simulink model "semaphore_0"  (R2024b)
settings: Solver=FixedStepDiscrete  StartTime=0.0  StopTime=inf  FixedStep=0.1  RelTol=1e-3
settings Model: PacingRate=0.040000  Creator=Gennaro  LastModifiedBy=miche
settings OptimizationCC: DefaultParameterBehavior=Inlined  UseDivisionForNetSlopeComputation=on  GainParamInheritBuiltInType=on  UseFloatMulNetSlope=on  InlineInvariantSignals=on  PassReuseOutputArgsAs=Individual arguments  ZeroExternalMemoryAtStartup=off  ZeroInternalMemoryAtStartup=off  NoFixptDivByZeroProtection=on  EfficientFloat2IntCast=on  LifeSpan=1  OptimizeBlockOrder=speed  DifferentSizesBufferReuse=on  EfficientTunableParamExpr=on
settings DebuggingCC: ParameterTunabilityLossMsg=error
settings HardwareCC: ProdBitPerPointer=32  ProdBitPerSizeT=32  ProdBitPerPtrDiffT=32  ProdLargestAtomicInteger=Long  ProdLargestAtomicFloat=Double  ProdWordSize=32  ProdLongLongMode=on  ProdHWDeviceType=ARM Compatible->ARM Cortex-M
settings SFSimCC: MATLABDynamicMemAlloc=off
settings RTWCC: Description=Embedded Coder  SystemTargetFile=ert.tlc  TemplateMakefile=ert_default_tmf
settings CodeAppCC: ForceParamTrailComments=on  IgnoreCustomStorageClasses=off  OperatorAnnotations=on  SimulinkDataObjDesc=on  SFDataObjDesc=on  CustomSymbolStrGlobalVar=rt$N$M  CustomSymbolStrType=$N$M  CustomSymbolStrFcn=$N$M$F  CustomSymbolStrMacro=$N$M  InsertBlockDesc=on
settings ERTTargetCC: TargetLangStandard=C99 (ISO)  GenerateSampleERTMain=on  IncludeMdlTerminateFcn=off  CombineSignalStateStructs=on  SupportAbsoluteTime=off  PurelyIntegerCode=on  SupportNonFinite=off  SupportComplex=off  SupportNonInlinedSFcns=on  ERTCustomFileTemplate=example_file_process.tlc  ERTFilePackagingFormat=CompactWithDataFile  DynamicArrayContainerType=coder::array

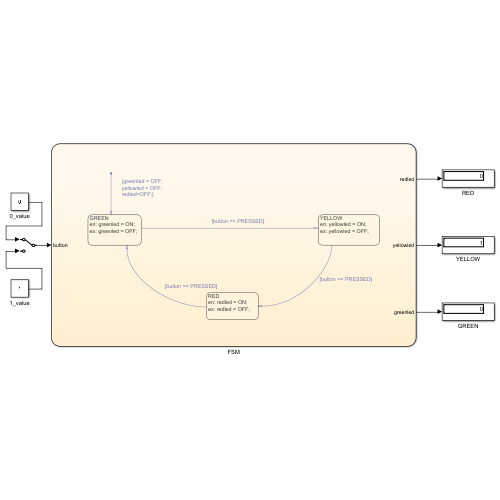
[thumbnail: Simulink's stored preview of the top-level diagram]
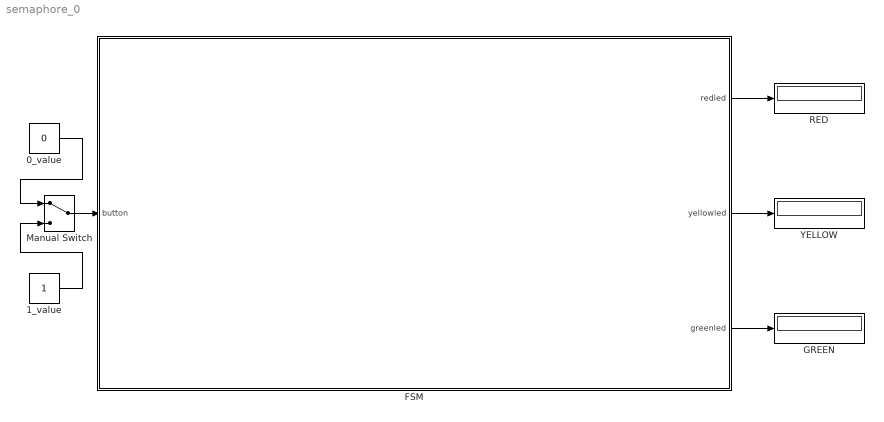
== system semaphore_0 ==
  0_value : Constant  Value=0  OutDataTypeStr=boolean
  1_value : Constant  OutDataTypeStr=boolean
  FSM : Stateflow chart  TreatAsAtomicUnit=on
  GREEN : Display
  Manual Switch : ManualSwitch
  RED : Display
  YELLOW : Display
  wires:
  Manual Switch/1 -> FSM/1(button)
  0_value/1 -> Manual Switch/1
  1_value/1 -> Manual Switch/2
  FSM/1(redled) -> RED/1
  FSM/2(yellowled) -> YELLOW/1
  FSM/3(greenled) -> GREEN/1

== stateflow chart semaphore_0/FSM ==
  state GREEN
    en: greenled = ON;
    ex: greenled = OFF;
  state YELLOW
    en: yellowled = ON;
    ex: yellowled = OFF;
  state RED
    en: redled = ON;
    ex: redled = OFF;
  (default) -> GREEN : {greenled = OFF;
      | yellowled = OFF;
      | redled=OFF;}
  GREEN -> YELLOW : [button == PRESSED]
  RED -> GREEN : [button == PRESSED]
  YELLOW -> RED : [button == PRESSED]
  data: button input boolean; PRESSED constant boolean =1; OFF constant boolean =0; ON constant boolean =1; redled output boolean; yellowled output boolean; greenled output boolean
